simulink model "air_quality"  (R2018b)
settings: Solver=VariableStepAuto  StartTime=0.0  StopTime=400  RelTol=1e-3
values from neighbouring files (symbols this model uses):
  stepsInDay = 24*60/timeStep    (= 288)    [init.m]
undefined symbols (not defined in the file or in its folder): bad_q, good_q
settings Model: Creator=Filipowicz_user1  LastModifiedBy=jf
settings SolverCC: ZeroCrossControl=DisableAll

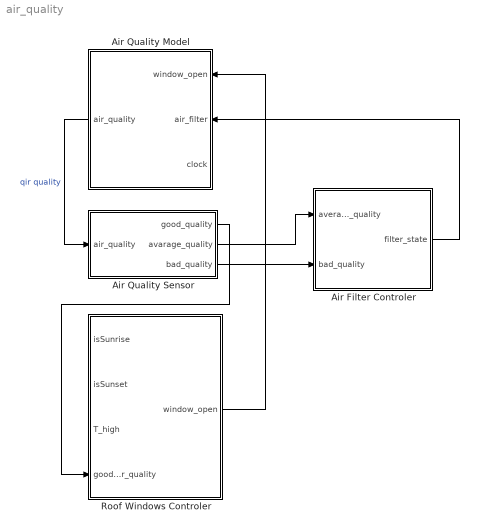
== system air_quality ==
  Air Filter Controler : Stateflow chart  TreatAsAtomicUnit=on
  Air Quality Model : Subsystem
  Air Quality Sensor : Subsystem
  Roof Windows Controler : Subsystem
  wires:
  Air Filter Controler/1(filter_state) -> Air Quality Model/2(air_filter)
  Air Quality Sensor/2(avarage_quality) -> Air Filter Controler/1(average_quality)
  Air Quality Sensor/3(bad_quality) -> Air Filter Controler/2(bad_quality)
  Air Quality Sensor/1(good_quality) -> Roof Windows Controler/4(good_air_quality)
  Roof Windows Controler/1(window_open) -> Air Quality Model/1(window_open)
  Air Quality Model/1(air_quality) -> Air Quality Sensor/1(air_quality)  "qir quality"

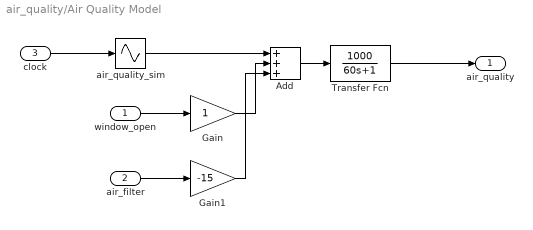
== system air_quality/Air Quality Model ==
  window_open : Inport
  air_filter : Inport  Port=2
  clock : Inport  Port=3
  Add : Sum  Inputs=+++
  Gain : Gain
  Gain1 : Gain  Gain=-15
  Transfer Fcn : TransferFcn  Numerator=[1000]  Denominator=[60 1]
  air_quality_sim : Sin  TimeSource=Use external signal  Amplitude=0.4  Bias=0.6  Frequency=2*pi/stepsInDay  Phase=-pi/2  SampleTime=0
  air_quality : Outport
  wires:
  Transfer Fcn/1 -> air_quality/1
  Gain/1 -> Add/2
  air_filter/1 -> Gain1/1
  Add/1 -> Transfer Fcn/1
  Gain1/1 -> Add/3
  air_quality_sim/1 -> Add/1
  window_open/1 -> Gain/1
  clock/1 -> air_quality_sim/1

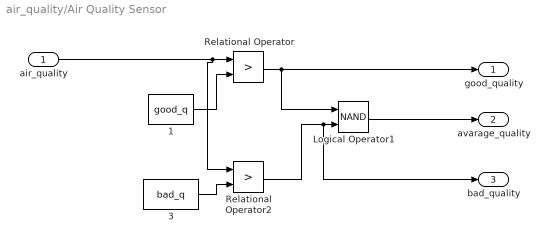
== system air_quality/Air Quality Sensor ==
  air_quality : Inport
  1 : Constant  Value=good_q
  3 : Constant  Value=bad_q
  Logical Operator1 : Logic  Operator=NAND  AllPortsSameDT=off  OutDataTypeStr=boolean
  Relational Operator : RelationalOperator  Operator=>  OutDataTypeStr=boolean  RndMeth=Simplest
  Relational Operator2 : RelationalOperator  Operator=>  OutDataTypeStr=boolean  RndMeth=Simplest
  good_quality : Outport
  avarage_quality : Outport  Port=2
  bad_quality : Outport  Port=3
  wires:
  3/1 -> Relational Operator2/2
  Relational Operator/1 -> Logical Operator1/1, good_quality/1
  1/1 -> Relational Operator/2
  Relational Operator2/1 -> Logical Operator1/2, bad_quality/1
  Logical Operator1/1 -> avarage_quality/1
  air_quality/1 -> Relational Operator/1, Relational Operator2/1

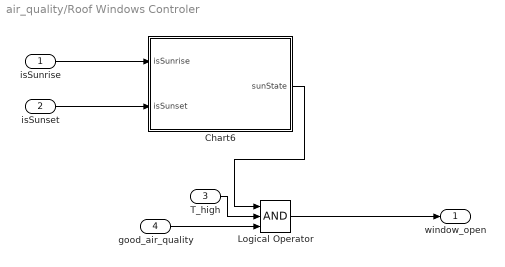
== system air_quality/Roof Windows Controler ==
  isSunrise : Inport
  isSunset : Inport  Port=2
  T_high : Inport  Port=3
  good_air_quality : Inport  Port=4
  Chart6 : Stateflow chart  TreatAsAtomicUnit=on
  Logical Operator : Logic  Inputs=3  AllPortsSameDT=off  OutDataTypeStr=boolean
  window_open : Outport
  wires:
  good_air_quality/1 -> Logical Operator/3
  T_high/1 -> Logical Operator/2
  Chart6/1(sunState) -> Logical Operator/1
  Logical Operator/1 -> window_open/1
  isSunset/1 -> Chart6/2(isSunset)
  isSunrise/1 -> Chart6/1(isSunrise)

== stateflow chart air_quality/Air Filter Controler ==
  state average
    filter_state=1;
  state good
    filter_state=0;
  (default) -> average
  average -> good : [average_quality]
  good -> average : [bad_quality]
  data: average_quality input; bad_quality input; filter_state output

== stateflow chart air_quality/Roof Windows Controler/Chart6 ==
  settings: updateMethod=DISCRETE  sampleTime=1  executeAtInitialization=1
  state sun_up
    sunState=false;
  state sun_down
    sunState=true;
  (default) -> sun_up
  sun_up -> sun_down : [isSunrise]
  sun_down -> sun_up : [isSunset]
  data: isSunrise input; isSunset input; sunState output
